simulink model "Junctions6_2018a"  (R2018a)
settings: Solver=FixedStepDiscrete  StartTime=0.0  StopTime=0.1  FixedStep=0.1  RelTol=1e-3  EnableMultiTasking=on
settings Model: Creator=BEAR  LastModifiedBy=bzhan
settings SolverCC: AutoInsertRateTranBlk=on
settings DataIOCC: LimitDataPoints=on
settings OptimizationCC: LifeSpan=inf
settings DebuggingCC: AllowSymbolicDim=off  SFUnexpectedBacktrackingDiag=warning  SFNoUnconditionalDefaultTransitionDiag=warning  SFExecutionAtInitializationDiag=none
settings CodeAppCC: StateflowObjectComments=on
settings GRTTargetCC: TargetLangStandard=C89/C90 (ANSI)
settings ConfigComp: CovMetricSettings=dw  CovHtmlReporting=on  CovSaveCumulativeToWorkspaceVar=on  CovSaveSingleToWorkspaceVar=on  CovShowResultsExplorer=off  CovExternalEMLEnable=off  CovSFcnEnable=off

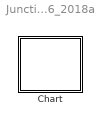
== system Junctions6_2018a ==
  Chart : Stateflow chart  TreatAsAtomicUnit=on

== stateflow chart Junctions6_2018a/Chart ==
  state A
    en: f("enA")
    ex: f("exA")
  state C
    en: f("enC")
    ex: f("exC")
  (default) -> A : {x=1;}
  A -> (junction 5) [order 1] : {x=-1;}/{f("ta1")}
  A -> (junction 5) [order 2] : {x=2;}/{f("ta2")}
  (junction 5) -> (junction 15) : {f("ca")}
  (junction 15) -> C : [x>0]/{f("ta4")}
  A -> (junction 5) [order 3] : {x=3;}/{f("ta3")}
  data: s function_input; x local
  function f(s):
    | function f(s)
    |     fprintf(s+"\n");
